simulink model "vfs_unity"  (R2022a)
settings: Solver=FixedStepAuto  StartTime=0.0  StopTime=inf  FixedStep=0.02  RelTol=1e-3
undefined symbols (not defined in the file): Angle, Angular, Axis, gd, gwc, Homogeneous, Kc, Linear, ros_freq, Rx, Ry, Rz, SE3, X, Y, Z
libraries: simlib_vpc_coremath x34, robotlib x25, simlib_vpc_basic x14, dspmtrx3 x5, simlib_vpc_gp x3
(part 2 of 2)

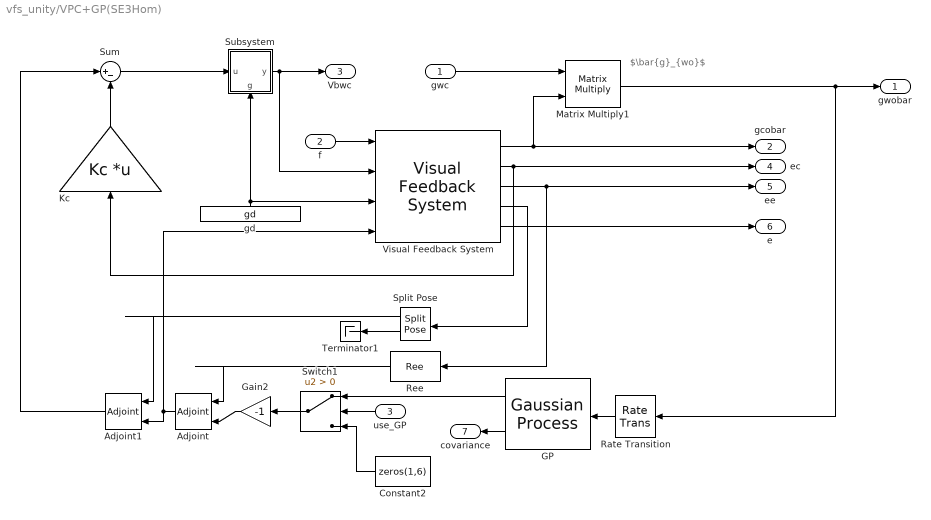
== system vfs_unity/VPC+GP(SE3Hom) ==
  note: $\bar{g}_{wo}$
  gwc : Inport
  f : Inport  Port=2
  use_GP : Inport  Port=3
  Adjoint : simlib_vpc_basic/Adjoint  adjointtype=orientation
      settings: SourceProductName=VPC Library
  Adjoint1 : simlib_vpc_basic/Adjoint  adjointtype=orientation
      settings: SourceProductName=VPC Library
  Constant2 : Constant  Value=zeros(1,6)
  GP : simlib_vpc_gp/Gaussian Process  X=X_GP_hom  Y=Y_GP_hom  sn=sn_GP_hom  kernel=SE3 (Homogeneous)  hyp=hyp_GP_hom  show_mean=on  show_variance=on  inv_fallback=off
      settings: SourceProductName=VPC Library
  Gain2 : Gain  Gain=-1
  Kc : Gain  Gain=Kc  Multiplication=Matrix(K*u) (u vector)
  Matrix Multiply1 : Product  Multiplication=Matrix(*)
  Rate Transition : RateTransition
  Ree : simlib_vpc_coremath/Ree
      settings: SourceProductName=VPC Library
  Split Pose : simlib_vpc_coremath/Split Pose  show_R=on  show_p=on
      settings: SourceProductName=VPC Library
  Subsystem : Subsystem
      settings: PortSchema="{\"entries\":[{\"content\":{\"sides\":[{\"content\":{\"connectorIds\":[\"In1\"]},\"type\":\"ConnectorPlacement.EquallySpacedRectSide\",\"uuid\":\"72e68008-5c4a-43a9-a560-64c6a31a0c08\"},{\"content\":{\"connectorIds\":[\"Out1\"],\"side\":\"RIGHT\"},\"type\":\"ConnectorPlacement.EquallySpacedRectSide\",\"uuid\":\"da07f5ff-2b2c-4c55-a2f2-34e133777503\"},{\"content\":{\"connectorIds\":[],\"side\":\"TOP\"},\"type\":\"ConnectorPlacement.EquallySpacedRectSide\",\"uuid\":\"6d174428-4364-4e89-aba7-4e9864808ab5\"},{\"content\":{\"connectorIds\":[\"In2\"],\"side\":\"BOTTOM\"},\"type\":\"ConnectorPlacement.EquallySpacedRectSide\",\"uuid\":\"f9633104-9c11-4d21-90a7-e0f886d9e92d\"},{\"content\":{\"connectorIds\":[],\"side\":\"HIDDEN\"},\"type\":\"ConnectorPlacement.EquallySpacedRectSide\",\"uuid\":\"662f08ae-9279-4a4f-85ea-81d97ead27d9\"}]},\"type\":\"ConnectorPlacement.EquallySpacedConnector\",\"uuid\":\"f3cd156c-cccd-47c6-b81c-6113f78efd58\"}],\"packageUris\":[\"http://schema.mathworks.com/mf0/Connector/R2020b\"],\"version\":\"1.0\"}"
      mask Display:
      | % Glitch in Matlab: If you define a line whose starting point and end point
      | % is equal, then the entire mask block is plotted in bold
      | plot([0,0],[0,0])
      | 
      | % Draw box
      | indent = 0.3;
      | ang=[0:0.2:pi/2, pi/2];
      | plot([0,1-indent],[0,0])
      | xp=indent*sin(ang)+1-indent;
      | yp=indent-indent*cos(ang);
      | plot(xp,yp);
      | plot([1,1,indent],[indent,1,1])
      | xp=indent-indent*sin(ang);
      | yp=1-indent+indent*cos(ang);
      | plot(xp,yp);
      | plot([0,0],[1-indent,0])
      | 
      | % Write label & ports
      | disp('-Ad_{(g_d)}','texmode','on')
      | text(0.5,0.2,'\fontsize{7}g_d','texmode','on')
  Sum : Sum  Inputs=|+-
  Switch1 : Switch  Criteria=u2 > Threshold  SaturateOnIntegerOverflow=off  InputSameDT=off
  Terminator1 : Terminator
  Visual Feedback System : simlib_vpc_basic/Visual Feedback System  gd_source=external  gd_value=[eye(4,3),ones(4,1)]  gcobar0=gco_init  Ke_source=internal  Ke=Ke  projection=on  camtype=Pinhole  fo=fp  lambda=lambda  show_Vbwo=off  show_ec=on  show_gce=on  show_ee=on  show_gee=off  show_e=on  show_nu=off  show_dgcobar=off  show_ue_aux=on
      settings: SourceProductName=VPC Library
  gd : Constant  Value=gd
  gwobar : Outport
  gcobar : Outport  Port=2
  Vbwc : Outport  Port=3
  ec : Outport  Port=4
  ee : Outport  Port=5
  e : Outport  Port=6
  covariance : Outport  Port=7
  wires:
  GP/1 -> Switch1/1
  Matrix Multiply1/1 -> Rate Transition/1, gwobar/1
  Visual Feedback System/4 -> Split Pose/1
  Adjoint1/1 -> Sum/1
  Sum/1 -> Subsystem/1(u)
  Switch1/1 -> Gain2/1
  Gain2/1 -> Adjoint/1
  Split Pose/2 -> Terminator1/1
  Ree/1 -> Adjoint/2
  Adjoint/1 -> Adjoint1/1, Visual Feedback System/4
  Rate Transition/1 -> GP/1
  Split Pose/1 -> Adjoint1/2
  Visual Feedback System/1 -> gcobar/1, Matrix Multiply1/2
  gd/1 -> Visual Feedback System/3, Subsystem/2(g)
  Visual Feedback System/3 -> ee/1, Ree/1
  Visual Feedback System/2 -> Kc/1, ec/1
  Kc/1 -> Sum/2
  Visual Feedback System/5 -> e/1
  gwc/1 -> Matrix Multiply1/1
  Subsystem/1(y) -> Visual Feedback System/2, Vbwc/1
  f/1 -> Visual Feedback System/1
  GP/2 -> covariance/1
  use_GP/1 -> Switch1/2
  Constant2/1 -> Switch1/3

== system vfs_unity/Standard/Subsystem ==
  u : Inport
  g : Inport  Port=2
  Adjoint : simlib_vpc_basic/Adjoint  adjointtype=pose
      settings: SourceProductName=VPC Library
  Gain : Gain  Gain=-1
  y : Outport
  wires:
  Adjoint/1 -> y/1
  u/1 -> Gain/1
  g/1 -> Adjoint/2
  Gain/1 -> Adjoint/1

== system vfs_unity/VPC+GP(SE)/Subsystem ==
  u : Inport
  g : Inport  Port=2
  Adjoint : simlib_vpc_basic/Adjoint  adjointtype=pose
      settings: SourceProductName=VPC Library
  Gain : Gain  Gain=-1
  y : Outport
  wires:
  Adjoint/1 -> y/1
  u/1 -> Gain/1
  g/1 -> Adjoint/2
  Gain/1 -> Adjoint/1

== system vfs_unity/VPC+GP(SE3Axang)/Subsystem ==
  u : Inport
  g : Inport  Port=2
  Adjoint : simlib_vpc_basic/Adjoint  adjointtype=pose
      settings: SourceProductName=VPC Library
  Gain : Gain  Gain=-1
  y : Outport
  wires:
  Adjoint/1 -> y/1
  u/1 -> Gain/1
  g/1 -> Adjoint/2
  Gain/1 -> Adjoint/1

== system vfs_unity/VPC+GP(SE3Hom)/Subsystem ==
  u : Inport
  g : Inport  Port=2
  Adjoint : simlib_vpc_basic/Adjoint  adjointtype=pose
      settings: SourceProductName=VPC Library
  Gain : Gain  Gain=-1
  y : Outport
  wires:
  Gain/1 -> Adjoint/1
  g/1 -> Adjoint/2
  u/1 -> Gain/1
  Adjoint/1 -> y/1

== matlab function vfs_unity/Agent4 Pose gwc/Convert Unity To Matlab ==
  data: vec_u input; vec_m output; rot input
function vec_m = unity2matlab(vec_u, rot) %#codegen
% Converts Unity coordinate system to Matlab system
%
% -----------
%
% Editor:
%   OMAINSKA Marco - Doctoral Student, Cybernetics
%       <marcoomainska@g.ecc.u-tokyo.ac.jp>
% Property of: Fujita-Yamauchi Lab, The University of Tokyo, 2022
% Website: https://www.scl.ipc.i.u-tokyo.ac.jp

%------------- BEGIN CODE --------------
vec_u = vec_u(:);

% define output dimension
vec_m = zeros(size(vec_u));

% transform to unity system
vec_m(1) = vec_u(1);
vec_m(2) = vec_u(3);
vec_m(3) = vec_u(2);
vec_m(4) = -vec_u(4);
vec_m(5) = -vec_u(6);
vec_m(6) = -vec_u(5);

% apply rot-transform if given
vec_m = adjoint(rot,'orientation') * vec_m;

%------------- END CODE --------------
end

== matlab function vfs_unity/Agent1 Pose gwc/Convert Unity To Matlab ==
  data: vec_u input; vec_m output; rot input
function vec_m = unity2matlab(vec_u, rot) %#codegen
% Converts Unity coordinate system to Matlab system
%
% -----------
%
% Editor:
%   OMAINSKA Marco - Doctoral Student, Cybernetics
%       <marcoomainska@g.ecc.u-tokyo.ac.jp>
% Property of: Fujita-Yamauchi Lab, The University of Tokyo, 2022
% Website: https://www.scl.ipc.i.u-tokyo.ac.jp

%------------- BEGIN CODE --------------
vec_u = vec_u(:);

% define output dimension
vec_m = zeros(size(vec_u));

% transform to unity system
vec_m(1) = vec_u(1);
vec_m(2) = vec_u(3);
vec_m(3) = vec_u(2);
vec_m(4) = -vec_u(4);
vec_m(5) = -vec_u(6);
vec_m(6) = -vec_u(5);

% apply rot-transform if given
vec_m = adjoint(rot,'orientation') * vec_m;

%------------- END CODE --------------
end

== matlab function vfs_unity/Set Target Estimate1/Convert Matlab To Unity ==
  data: vec_m input; vec_u output; rot input
function vec_u = matlab2unity(vec_m, rot) %#codegen
% Converts Matlab coordinate system to Unity system
%
% -----------
%
% Editor:
%   OMAINSKA Marco - Doctoral Student, Cybernetics
%       <marcoomainska@g.ecc.u-tokyo.ac.jp>
% Property of: Fujita-Yamauchi Lab, The University of Tokyo, 2022
% Website: https://www.scl.ipc.i.u-tokyo.ac.jp

%------------- BEGIN CODE --------------
vec_m = vec_m(:);

% define output dimension
vec_u = zeros(size(vec_m));

% apply rot-transform if given
vec_m = adjoint(rot,'orientation') * vec_m;

% transform to unity system
vec_u(1) = vec_m(1);
vec_u(2) = vec_m(3);
vec_u(3) = vec_m(2);
vec_u(4) = -vec_m(4);
vec_u(5) = -vec_m(6);
vec_u(6) = -vec_m(5);

%------------- END CODE --------------
end

== matlab function vfs_unity/Target Pose gwo/Convert Unity To Matlab ==
  data: vec_u input; vec_m output; rot input
function vec_m = unity2matlab(vec_u, rot) %#codegen
% Converts Unity coordinate system to Matlab system
%
% -----------
%
% Editor:
%   OMAINSKA Marco - Doctoral Student, Cybernetics
%       <marcoomainska@g.ecc.u-tokyo.ac.jp>
% Property of: Fujita-Yamauchi Lab, The University of Tokyo, 2022
% Website: https://www.scl.ipc.i.u-tokyo.ac.jp

%------------- BEGIN CODE --------------
vec_u = vec_u(:);

% define output dimension
vec_m = zeros(size(vec_u));

% transform to unity system
vec_m(1) = vec_u(1);
vec_m(2) = vec_u(3);
vec_m(3) = vec_u(2);
vec_m(4) = -vec_u(4);
vec_m(5) = -vec_u(6);
vec_m(6) = -vec_u(5);

% apply rot-transform if given
vec_m = adjoint(rot,'orientation') * vec_m;

%------------- END CODE --------------
end

== matlab function vfs_unity/Agent2 Pose gwc/Convert Unity To Matlab ==
  data: vec_u input; vec_m output; rot input
function vec_m = unity2matlab(vec_u, rot) %#codegen
% Converts Unity coordinate system to Matlab system
%
% -----------
%
% Editor:
%   OMAINSKA Marco - Doctoral Student, Cybernetics
%       <marcoomainska@g.ecc.u-tokyo.ac.jp>
% Property of: Fujita-Yamauchi Lab, The University of Tokyo, 2022
% Website: https://www.scl.ipc.i.u-tokyo.ac.jp

%------------- BEGIN CODE --------------
vec_u = vec_u(:);

% define output dimension
vec_m = zeros(size(vec_u));

% transform to unity system
vec_m(1) = vec_u(1);
vec_m(2) = vec_u(3);
vec_m(3) = vec_u(2);
vec_m(4) = -vec_u(4);
vec_m(5) = -vec_u(6);
vec_m(6) = -vec_u(5);

% apply rot-transform if given
vec_m = adjoint(rot,'orientation') * vec_m;

%------------- END CODE --------------
end

== matlab function vfs_unity/Agent3 Pose gwc/Convert Unity To Matlab ==
  data: vec_u input; vec_m output; rot input
function vec_m = unity2matlab(vec_u, rot) %#codegen
% Converts Unity coordinate system to Matlab system
%
% -----------
%
% Editor:
%   OMAINSKA Marco - Doctoral Student, Cybernetics
%       <marcoomainska@g.ecc.u-tokyo.ac.jp>
% Property of: Fujita-Yamauchi Lab, The University of Tokyo, 2022
% Website: https://www.scl.ipc.i.u-tokyo.ac.jp

%------------- BEGIN CODE --------------
vec_u = vec_u(:);

% define output dimension
vec_m = zeros(size(vec_u));

% transform to unity system
vec_m(1) = vec_u(1);
vec_m(2) = vec_u(3);
vec_m(3) = vec_u(2);
vec_m(4) = -vec_u(4);
vec_m(5) = -vec_u(6);
vec_m(6) = -vec_u(5);

% apply rot-transform if given
vec_m = adjoint(rot,'orientation') * vec_m;

%------------- END CODE --------------
end

== matlab function vfs_unity/Agent2 Cmd_vel/Convert Matlab To Unity ==
  data: vec_m input; vec_u output; rot input
function vec_u = matlab2unity(vec_m, rot) %#codegen
% Converts Matlab coordinate system to Unity system
%
% -----------
%
% Editor:
%   OMAINSKA Marco - Doctoral Student, Cybernetics
%       <marcoomainska@g.ecc.u-tokyo.ac.jp>
% Property of: Fujita-Yamauchi Lab, The University of Tokyo, 2022
% Website: https://www.scl.ipc.i.u-tokyo.ac.jp

%------------- BEGIN CODE --------------
vec_m = vec_m(:);

% define output dimension
vec_u = zeros(size(vec_m));

% apply rot-transform if given
vec_m = adjoint(rot,'orientation') * vec_m;

% transform to unity system
vec_u(1) = vec_m(1);
vec_u(2) = vec_m(3);
vec_u(3) = vec_m(2);
vec_u(4) = -vec_m(4);
vec_u(5) = -vec_m(6);
vec_u(6) = -vec_m(5);

%------------- END CODE --------------
end

== matlab function vfs_unity/Set Target Estimate2/Convert Matlab To Unity ==
  data: vec_m input; vec_u output; rot input
function vec_u = matlab2unity(vec_m, rot) %#codegen
% Converts Matlab coordinate system to Unity system
%
% -----------
%
% Editor:
%   OMAINSKA Marco - Doctoral Student, Cybernetics
%       <marcoomainska@g.ecc.u-tokyo.ac.jp>
% Property of: Fujita-Yamauchi Lab, The University of Tokyo, 2022
% Website: https://www.scl.ipc.i.u-tokyo.ac.jp

%------------- BEGIN CODE --------------
vec_m = vec_m(:);

% define output dimension
vec_u = zeros(size(vec_m));

% apply rot-transform if given
vec_m = adjoint(rot,'orientation') * vec_m;

% transform to unity system
vec_u(1) = vec_m(1);
vec_u(2) = vec_m(3);
vec_u(3) = vec_m(2);
vec_u(4) = -vec_m(4);
vec_u(5) = -vec_m(6);
vec_u(6) = -vec_m(5);

%------------- END CODE --------------
end

== matlab function vfs_unity/Agent3 Cmd_vel/Convert Matlab To Unity ==
  data: vec_m input; vec_u output; rot input
function vec_u = matlab2unity(vec_m, rot) %#codegen
% Converts Matlab coordinate system to Unity system
%
% -----------
%
% Editor:
%   OMAINSKA Marco - Doctoral Student, Cybernetics
%       <marcoomainska@g.ecc.u-tokyo.ac.jp>
% Property of: Fujita-Yamauchi Lab, The University of Tokyo, 2022
% Website: https://www.scl.ipc.i.u-tokyo.ac.jp

%------------- BEGIN CODE --------------
vec_m = vec_m(:);

% define output dimension
vec_u = zeros(size(vec_m));

% apply rot-transform if given
vec_m = adjoint(rot,'orientation') * vec_m;

% transform to unity system
vec_u(1) = vec_m(1);
vec_u(2) = vec_m(3);
vec_u(3) = vec_m(2);
vec_u(4) = -vec_m(4);
vec_u(5) = -vec_m(6);
vec_u(6) = -vec_m(5);

%------------- END CODE --------------
end

== matlab function vfs_unity/Agent1 Cmd_vel/Convert Matlab To Unity ==
  data: vec_m input; vec_u output; rot input
function vec_u = matlab2unity(vec_m, rot) %#codegen
% Converts Matlab coordinate system to Unity system
%
% -----------
%
% Editor:
%   OMAINSKA Marco - Doctoral Student, Cybernetics
%       <marcoomainska@g.ecc.u-tokyo.ac.jp>
% Property of: Fujita-Yamauchi Lab, The University of Tokyo, 2022
% Website: https://www.scl.ipc.i.u-tokyo.ac.jp

%------------- BEGIN CODE --------------
vec_m = vec_m(:);

% define output dimension
vec_u = zeros(size(vec_m));

% apply rot-transform if given
vec_m = adjoint(rot,'orientation') * vec_m;

% transform to unity system
vec_u(1) = vec_m(1);
vec_u(2) = vec_m(3);
vec_u(3) = vec_m(2);
vec_u(4) = -vec_m(4);
vec_u(5) = -vec_m(6);
vec_u(6) = -vec_m(5);

%------------- END CODE --------------
end

== matlab function vfs_unity/Set Target Estimate3/Convert Matlab To Unity ==
  data: vec_m input; vec_u output; rot input
function vec_u = matlab2unity(vec_m, rot) %#codegen
% Converts Matlab coordinate system to Unity system
%
% -----------
%
% Editor:
%   OMAINSKA Marco - Doctoral Student, Cybernetics
%       <marcoomainska@g.ecc.u-tokyo.ac.jp>
% Property of: Fujita-Yamauchi Lab, The University of Tokyo, 2022
% Website: https://www.scl.ipc.i.u-tokyo.ac.jp

%------------- BEGIN CODE --------------
vec_m = vec_m(:);

% define output dimension
vec_u = zeros(size(vec_m));

% apply rot-transform if given
vec_m = adjoint(rot,'orientation') * vec_m;

% transform to unity system
vec_u(1) = vec_m(1);
vec_u(2) = vec_m(3);
vec_u(3) = vec_m(2);
vec_u(4) = -vec_m(4);
vec_u(5) = -vec_m(6);
vec_u(6) = -vec_m(5);

%------------- END CODE --------------
end

== matlab function vfs_unity/Agent4 Cmd_vel/Convert Matlab To Unity ==
  data: vec_m input; vec_u output; rot input
function vec_u = matlab2unity(vec_m, rot) %#codegen
% Converts Matlab coordinate system to Unity system
%
% -----------
%
% Editor:
%   OMAINSKA Marco - Doctoral Student, Cybernetics
%       <marcoomainska@g.ecc.u-tokyo.ac.jp>
% Property of: Fujita-Yamauchi Lab, The University of Tokyo, 2022
% Website: https://www.scl.ipc.i.u-tokyo.ac.jp

%------------- BEGIN CODE --------------
vec_m = vec_m(:);

% define output dimension
vec_u = zeros(size(vec_m));

% apply rot-transform if given
vec_m = adjoint(rot,'orientation') * vec_m;

% transform to unity system
vec_u(1) = vec_m(1);
vec_u(2) = vec_m(3);
vec_u(3) = vec_m(2);
vec_u(4) = -vec_m(4);
vec_u(5) = -vec_m(6);
vec_u(6) = -vec_m(5);

%------------- END CODE --------------
end

== matlab function vfs_unity/Set Target Estimate4/Convert Matlab To Unity ==
  data: vec_m input; vec_u output; rot input
function vec_u = matlab2unity(vec_m, rot) %#codegen
% Converts Matlab coordinate system to Unity system
%
% -----------
%
% Editor:
%   OMAINSKA Marco - Doctoral Student, Cybernetics
%       <marcoomainska@g.ecc.u-tokyo.ac.jp>
% Property of: Fujita-Yamauchi Lab, The University of Tokyo, 2022
% Website: https://www.scl.ipc.i.u-tokyo.ac.jp

%------------- BEGIN CODE --------------
vec_m = vec_m(:);

% define output dimension
vec_u = zeros(size(vec_m));

% apply rot-transform if given
vec_m = adjoint(rot,'orientation') * vec_m;

% transform to unity system
vec_u(1) = vec_m(1);
vec_u(2) = vec_m(3);
vec_u(3) = vec_m(2);
vec_u(4) = -vec_m(4);
vec_u(5) = -vec_m(6);
vec_u(6) = -vec_m(5);

%------------- END CODE --------------
end
